simulink model "gm_sampleModel1911_sub_sub"  (R2023a)
settings: Solver=VariableStepAuto  StartTime=0.0  StopTime=10.0  RelTol=1e-3
libraries: simulink x3, hdlsllib x2
settings Model: Creator=user1  LastModifiedBy=user1
settings OptimizationCC: BlockReduction=off  ConditionallyExecuteInputs=off
settings DebuggingCC: InheritedTsInSrcMsg=none

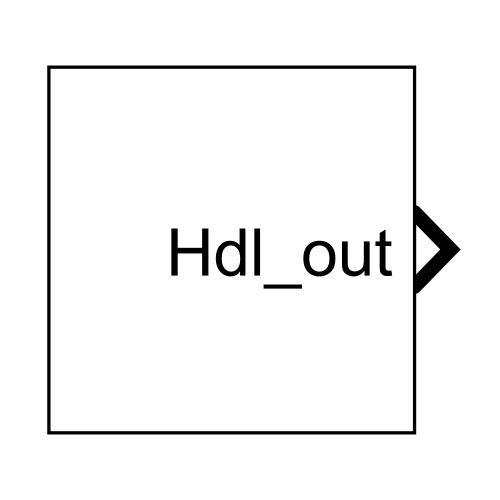
[thumbnail: Simulink's stored preview of the top-level diagram]
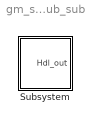
== system gm_sampleModel1911_sub_sub ==
  Subsystem : Subsystem

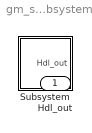
== system gm_sampleModel1911_sub_sub/Subsystem ==
  Subsystem : Subsystem
  Hdl_out : Outport  OutDataTypeStr=uint8

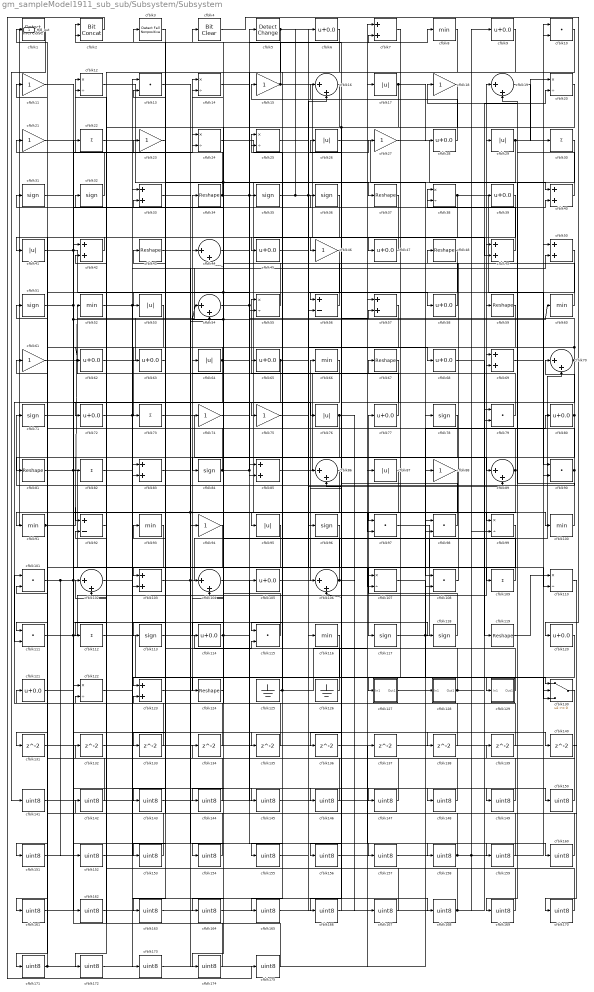
== system gm_sampleModel1911_sub_sub/Subsystem/Subsystem ==
  cfblk1 : simulink/Logic and Bit Operations/Detect Increase  vinit=0.0  OutDataTypeStr=uint8
      settings: LibrarySourceBlock=|
      | hdlsllib/Logic and Bit
      | Operations/Detect
      | Increase
  cfblk{10,13,79,90,97..98,101,108,111,115} (10 alike) : DotProduct  OutDataTypeStr=uint8
  cfblk{8,52,60,66,91,93,100,116} (8 alike) : MinMax  OutDataTypeStr=uint8
  cfblk{16,19,44,54,70,86,89,102,104,106} (10 alike) : Sum  Inputs=|++  OutDataTypeStr=uint8
  cfblk{7,33,40,42,49..50,57,69,83,85,103,123} (12 alike) : Sum  OutDataTypeStr=uint8
  cfblk{6,9,28,39,45,47,58,62..63,65,68,72,77,80,105,114,120..121} (18 alike) : Bias  Bias=0.0  SaturateOnIntegerOverflow=off
  cfblk{12,14,20,24..25,38,55,99,107,110,122} (11 alike) : Product  Inputs=*/  OutDataTypeStr=uint8  RndMeth=Zero  SaturateOnIntegerOverflow=on
  cfblk{22,30,73,82,109,112} (6 alike) : Sum  Inputs=+  OutDataTypeStr=uint8
  cfblk{11,15,18,21,23,27,46,61,74..75,88,94} (12 alike) : Gain  OutDataTypeStr=uint8
  cfblk{31..32,35..36,51,71,78,84,96,113,117..118} (12 alike) : Signum
  cfblk{34,37,43,48,59,67,81,119,124} (9 alike) : Reshape
  cfblk125 : Ground
  cfblk126 : Ground
  cfblk127 : Subsystem
      settings: LibrarySourceBlock=|
      | hdlsllib/Ports &
      | Subsystems/Subsystem
  cfblk128 : Subsystem
      settings: LibrarySourceBlock=|
      | hdlsllib/Ports &
      | Subsystems/Subsystem
  cfblk129 : Subsystem
      settings: LibrarySourceBlock=|
      | hdlsllib/Ports &
      | Subsystems/Subsystem
  cfblk130 : Switch  OutDataTypeStr=uint8  SaturateOnIntegerOverflow=off  InputSameDT=off
  cfblk{131..140} (10 alike) : Delay  SampleTime=1
  cfblk{141..175} (35 alike) : DataTypeConversion  OutDataTypeStr=uint8  SaturateOnIntegerOverflow=off  RndMeth=Floor
  cfblk{17,26,29,41,53,64,76,87,95} (9 alike) : Abs  OutDataTypeStr=uint8  SaturateOnIntegerOverflow=off
  cfblk2 : hdlsllib/Logic and Bit Operations/Bit Concat  numInputs=2
  cfblk3 : hdlsllib/Logic and Bit Operations/Detect Fall Nonpositive  vinit=0  OutDataTypeStr=uint8
  cfblk4 : simulink/Logic and Bit Operations/Bit Clear  iBit=0
      settings: LibrarySourceBlock=|
      | hdlsllib/Logic and Bit
      | Operations/Bit Clear
  cfblk5 : simulink/Logic and Bit Operations/Detect Change  vinit=0  OutDataTypeStr=uint8
      settings: LibrarySourceBlock=|
      | hdlsllib/Logic and Bit
      | Operations/Detect
      | Change
  cfblk56 : Sum  Inputs=+-  OutDataTypeStr=uint8
  cfblk92 : Sum  Inputs=+-  OutDataTypeStr=uint8
  Hdl_out : Outport  OutDataTypeStr=uint8
  wires:
  cfblk89/1 -> cfblk166/1, cfblk19/1
  cfblk35/1 -> cfblk6/1, cfblk49/2, cfblk47/1
  cfblk40/1 -> cfblk19/2
  cfblk53/1 -> cfblk73/1
  cfblk119/1 -> cfblk110/1
  cfblk90/1 -> cfblk42/2, cfblk71/1
  cfblk123/1 -> cfblk34/1
  cfblk22/1 -> cfblk46/1
  cfblk106/1 -> cfblk137/1, cfblk24/1
  cfblk18/1 -> cfblk56/1
  cfblk97/1 -> cfblk110/2
  cfblk55/1 -> cfblk21/1
  cfblk48/1 -> cfblk53/1
  cfblk92/1 -> cfblk32/1
  cfblk56/1 -> cfblk2/1
  cfblk80/1 -> cfblk84/1, cfblk70/1
  cfblk34/1 -> cfblk14/2, cfblk147/1, cfblk98/2
  cfblk88/1 -> cfblk171/1
  cfblk47/1 -> cfblk45/1
  cfblk108/1 -> cfblk48/1
  cfblk84/1 -> cfblk51/1, cfblk140/1, cfblk38/2
  cfblk105/1 -> cfblk66/1
  cfblk54/1 -> cfblk57/2, cfblk5/1
  cfblk42/1 -> cfblk41/1
  cfblk77/1 -> cfblk55/1
  cfblk8/1 -> cfblk75/1
  cfblk19/1 -> cfblk30/1
  cfblk98/1 -> cfblk4/1
  cfblk117/1 -> cfblk80/1, cfblk29/1
  cfblk76/1 -> cfblk167/1, cfblk151/1
  cfblk63/1 -> cfblk43/1
  cfblk39/1 -> cfblk81/1
  cfblk91/1 -> Hdl_out/1, cfblk52/1
  cfblk69/1 -> cfblk50/1
  cfblk85/1 -> cfblk7/1
  cfblk15/1 -> cfblk2/2, cfblk78/1
  cfblk66/1 -> cfblk91/1
  cfblk103/1 -> cfblk50/2, cfblk70/2
  cfblk28/1 -> cfblk15/1
  cfblk9/1 -> cfblk72/1
  cfblk32/1 -> cfblk12/1
  cfblk6/1 -> cfblk55/2
  cfblk72/1 -> cfblk129/1(In1), cfblk67/1
  cfblk111/1 -> cfblk157/1, cfblk59/1
  cfblk27/1 -> cfblk40/1
  cfblk49/1 -> cfblk38/1
  cfblk12/1 -> cfblk37/1
  cfblk38/1 -> cfblk127/1(In1), cfblk90/1
  cfblk33/1 -> cfblk158/1
  cfblk81/1 -> cfblk99/1, cfblk117/1
  cfblk44/1 -> cfblk8/1
  cfblk71/1 -> cfblk118/1
  cfblk37/1 -> cfblk95/1
  cfblk100/1 -> cfblk18/1
  cfblk127/1(Out1) -> cfblk128/1(In1)
  cfblk60/1 -> cfblk25/1
  cfblk70/1 -> cfblk156/1, cfblk62/1, cfblk26/1
  cfblk118/1 -> cfblk77/1
  cfblk112/1 -> cfblk130/1
  cfblk87/1 -> cfblk112/1
  cfblk58/1 -> cfblk14/1
  cfblk125/1 -> cfblk87/1, cfblk65/1
  cfblk36/1 -> cfblk113/1
  cfblk41/1 -> cfblk109/1, cfblk85/1
  cfblk121/1 -> cfblk60/1, cfblk36/1
  cfblk29/1 -> cfblk20/1, cfblk154/1, cfblk103/1
  cfblk52/1 -> cfblk49/1, cfblk100/1
  cfblk73/1 -> cfblk89/1
  cfblk124/1 -> cfblk64/1
  cfblk20/1 -> cfblk115/1
  cfblk17/1 -> cfblk28/1, cfblk106/2, cfblk104/2
  cfblk14/1 -> cfblk7/2
  cfblk101/1 -> cfblk152/1, cfblk149/1, cfblk24/2
  cfblk74/1 -> cfblk40/2
  cfblk102/1 -> cfblk168/1
  cfblk113/1 -> cfblk115/2
  cfblk78/1 -> cfblk92/1
  cfblk26/1 -> cfblk108/1
  cfblk79/1 -> cfblk69/1
  cfblk107/1 -> cfblk130/2
  cfblk7/1 -> cfblk107/1
  cfblk43/1 -> cfblk138/1, cfblk97/2
  cfblk65/1 -> cfblk111/2, cfblk107/2
  cfblk62/1 -> cfblk44/1
  cfblk129/1(Out1) -> cfblk93/1
  cfblk45/1 -> cfblk68/1
  cfblk51/1 -> cfblk76/1, cfblk22/1
  cfblk120/1 -> cfblk124/1
  cfblk24/1 -> cfblk27/1
  cfblk5/1 -> cfblk89/2, cfblk85/2
  cfblk128/1(Out1) -> cfblk20/2, cfblk16/1
  cfblk115/1 -> cfblk31/1
  cfblk82/1 -> cfblk97/1
  cfblk109/1 -> cfblk25/2
  cfblk126/1 -> cfblk54/1, cfblk44/2
  cfblk46/1 -> cfblk111/1, cfblk114/1
  cfblk114/1 -> cfblk74/1, cfblk130/3
  cfblk4/1 -> cfblk120/1
  cfblk96/1 -> cfblk123/1
  cfblk25/1 -> cfblk58/1
  cfblk68/1 -> cfblk119/1
  cfblk61/1 -> cfblk69/2, cfblk35/1
  cfblk75/1 -> cfblk16/2
  cfblk93/1 -> cfblk103/2
  cfblk64/1 -> cfblk146/1, cfblk82/1, cfblk63/1
  cfblk57/1 -> cfblk131/1
  cfblk131/1 -> cfblk56/2
  cfblk132/1 -> cfblk90/2
  cfblk50/1 -> cfblk133/1
  cfblk133/1 -> cfblk92/2
  cfblk130/1 -> cfblk134/1
  cfblk134/1 -> cfblk42/1
  cfblk31/1 -> cfblk135/1
  cfblk135/1 -> cfblk12/2
  cfblk67/1 -> cfblk136/1
  cfblk137/1 -> cfblk98/1
  cfblk138/1 -> cfblk104/1
  cfblk139/1 -> cfblk101/1
  cfblk1/1 -> cfblk141/1
  cfblk141/1 -> cfblk17/1
  cfblk140/1 -> cfblk142/1
  cfblk142/1 -> cfblk1/1
  cfblk3/1 -> cfblk143/1
  cfblk143/1 -> cfblk105/1
  cfblk95/1 -> cfblk144/1
  cfblk144/1 -> cfblk3/1
  cfblk13/1 -> cfblk145/1
  cfblk145/1 -> cfblk106/1
  cfblk146/1 -> cfblk13/1
  cfblk147/1 -> cfblk13/2
  cfblk11/1 -> cfblk148/1
  cfblk148/1 -> cfblk61/1
  cfblk149/1 -> cfblk11/1
  cfblk83/1 -> cfblk150/1
  cfblk150/1 -> cfblk139/1
  cfblk151/1 -> cfblk83/1
  cfblk152/1 -> cfblk83/2
  cfblk23/1 -> cfblk153/1
  cfblk153/1 -> cfblk101/2
  cfblk154/1 -> cfblk23/1
  cfblk10/1 -> cfblk155/1
  cfblk155/1 -> cfblk96/1
  cfblk156/1 -> cfblk10/1
  cfblk157/1 -> cfblk10/2
  cfblk158/1 -> cfblk123/2, cfblk9/1, cfblk39/1
  cfblk136/1 -> cfblk159/1
  cfblk159/1 -> cfblk33/1
  cfblk104/1 -> cfblk160/1
  cfblk160/1 -> cfblk33/2
  cfblk94/1 -> cfblk161/1
  cfblk161/1 -> cfblk108/2
  cfblk21/1 -> cfblk162/1
  cfblk162/1 -> cfblk94/1
  cfblk116/1 -> cfblk163/1
  cfblk163/1 -> cfblk79/1
  cfblk59/1 -> cfblk164/1
  cfblk164/1 -> cfblk116/1
  cfblk86/1 -> cfblk165/1
  cfblk165/1 -> cfblk79/2
  cfblk166/1 -> cfblk86/1
  cfblk167/1 -> cfblk86/2
  cfblk168/1 -> cfblk99/2, cfblk132/1
  cfblk30/1 -> cfblk169/1
  cfblk169/1 -> cfblk102/1
  cfblk110/1 -> cfblk170/1
  cfblk170/1 -> cfblk102/2
  cfblk171/1 -> cfblk121/1, cfblk54/2
  cfblk16/1 -> cfblk172/1
  cfblk172/1 -> cfblk88/1
  cfblk122/1 -> cfblk173/1
  cfblk173/1 -> cfblk57/1
  cfblk99/1 -> cfblk174/1
  cfblk174/1 -> cfblk122/1
  cfblk2/1 -> cfblk175/1
  cfblk175/1 -> cfblk122/2

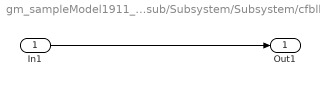
== system gm_sampleModel1911_sub_sub/Subsystem/Subsystem/cfblk127 ==
  In1 : Inport
  Out1 : Outport
  wires:
  In1/1 -> Out1/1

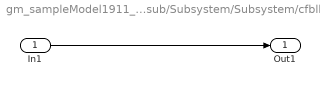
== system gm_sampleModel1911_sub_sub/Subsystem/Subsystem/cfblk128 ==
  In1 : Inport
  Out1 : Outport
  wires:
  In1/1 -> Out1/1

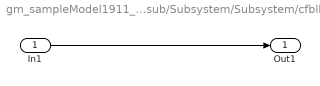
== system gm_sampleModel1911_sub_sub/Subsystem/Subsystem/cfblk129 ==
  In1 : Inport
  Out1 : Outport
  wires:
  In1/1 -> Out1/1
